simulink model "RLC_circuit"  (R2019b)
settings: Solver=VariableStepAuto  StartTime=0.0  StopTime=10.0  RelTol=1e-3
undefined symbols (not defined in the file or in its folder): l
settings Model: Creator=bhanu prasad  LastModifiedBy=bhanu prasad

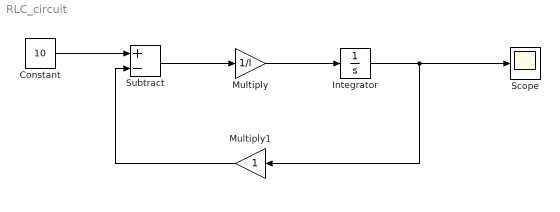
== system RLC_circuit ==
  Constant : Constant  Value=10
  Integrator : Integrator
  Multiply : Gain  Gain=1/l
  Multiply1 : Gain
  Scope : Scope
  Subtract : Sum  Inputs=+-
  wires:
  Constant/1 -> Subtract/1
  Subtract/1 -> Multiply/1
  Multiply/1 -> Integrator/1
  Integrator/1 -> Scope/1, Multiply1/1
  Multiply1/1 -> Subtract/2
